simulink model "Simulink_carro"  (R2025b)
settings: Solver=VariableStepAuto  StartTime=0.0  StopTime=10.0  RelTol=1e-3
settings Model: Creator=lhyul  LastModifiedBy=lhyul

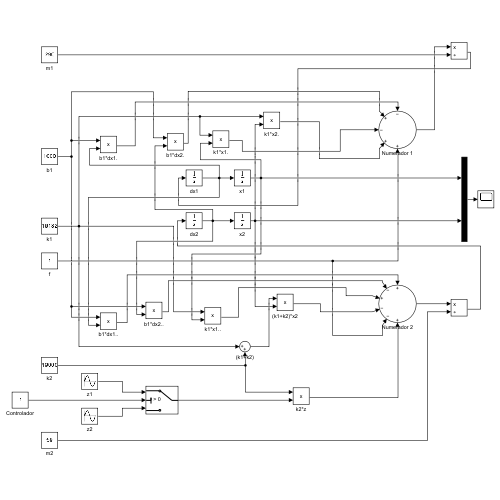
[thumbnail: Simulink's stored preview of the top-level diagram]
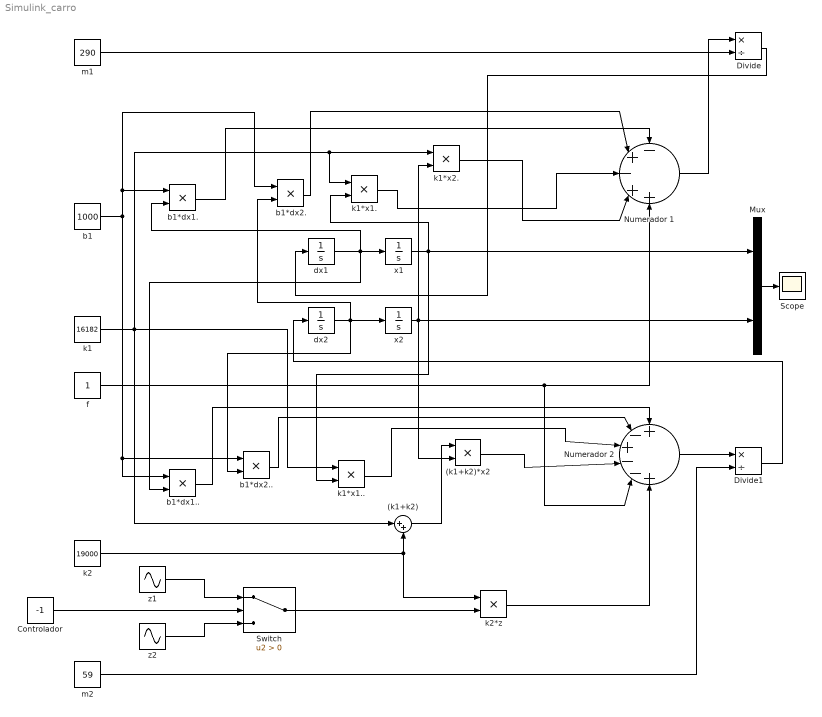
== system Simulink_carro ==
  (k1+k2) : Sum  Inputs=|++
  (k1+k2)*x2 : Product
  Controlador : Constant  Value=-1
  Divide : Product  Inputs=*/
  Divide1 : Product  Inputs=*/
  Mux : Mux  Inputs=2
  Numerador 1 : Sum  Inputs=-+-++
  Numerador 2 : Sum  Inputs=+-+--+
  Scope : Scope
      settings: ActiveDisplayYMinimum=-0.0083261559120885228  ActiveDisplayYMaximum=0.013651196014192185
  Switch : Switch  Criteria=u2 > Threshold  SaturateOnIntegerOverflow=off  InputSameDT=off
  b1 : Constant  Value=1000
  b1*dx1. : Product
  b1*dx1.. : Product
  b1*dx2. : Product
  b1*dx2.. : Product
  dx1 : Integrator
  dx2 : Integrator
  f : Constant
  k1 : Constant  Value=16182
  k1*x1. : Product
  k1*x1.. : Product
  k1*x2. : Product
  k2 : Constant  Value=19000
  k2*z : Product
  m1 : Constant  Value=290
  m2 : Constant  Value=59
  x1 : Integrator
  x2 : Integrator
  z1 : Sin  Amplitude=0.05  Frequency=0.5*pi  SampleTime=0
  z2 : Sin  Amplitude=0.05  Frequency=20*pi  SampleTime=0
  wires:
  dx1/1 -> b1*dx1./2, b1*dx1../2, x1/1
  dx2/1 -> x2/1, b1*dx2../2, b1*dx2./2
  b1/1 -> b1*dx2./1, b1*dx1./1, b1*dx2../1, b1*dx1../1
  x1/1 -> k1*x1../2, Mux/1, k1*x1./2
  k1/1 -> k1*x1./1, k1*x2./1, k1*x1../1, (k1+k2)/1
  x2/1 -> k1*x2./2, Mux/2, (k1+k2)*x2/2
  b1*dx1./1 -> Numerador 1/1
  b1*dx2./1 -> Numerador 1/2
  k1*x1./1 -> Numerador 1/3
  k1*x2./1 -> Numerador 1/4
  f/1 -> Numerador 1/5, Numerador 2/5
  k2/1 -> k2*z/1, (k1+k2)/2
  (k1+k2)/1 -> (k1+k2)*x2/1
  z1/1 -> Switch/1
  z2/1 -> Switch/3
  Switch/1 -> k2*z/2
  Controlador/1 -> Switch/2
  b1*dx1../1 -> Numerador 2/1
  b1*dx2../1 -> Numerador 2/2
  k1*x1../1 -> Numerador 2/3
  (k1+k2)*x2/1 -> Numerador 2/4
  k2*z/1 -> Numerador 2/6
  Numerador 1/1 -> Divide/1
  m1/1 -> Divide/2
  Numerador 2/1 -> Divide1/1
  m2/1 -> Divide1/2
  Divide/1 -> dx1/1
  Divide1/1 -> dx2/1
  Mux/1 -> Scope/1
